simulink model "ex1"  (R2015a)
settings: Solver=ode45  StartTime=0.0  StopTime=10.0  RelTol=1e-3
values from neighbouring files (symbols this model uses):
  Nfft = 128    [e1.m]
  Ng = 16    [e1.m]
  Nsym = Nfft+Ng    (= 144)    [e1.m]
undefined symbols (not defined in the file or in its folder): get, magnitude
libraries: dspxfrm3 x2, dspindex x2, commdigbbndam3 x2, dspsnks4 x2, dspstat3 x2, commchan3 x1, commrandsrc2 x1, commsink2 x1, simulink x1
settings Model: Creator=david  LastModifiedBy=ctu

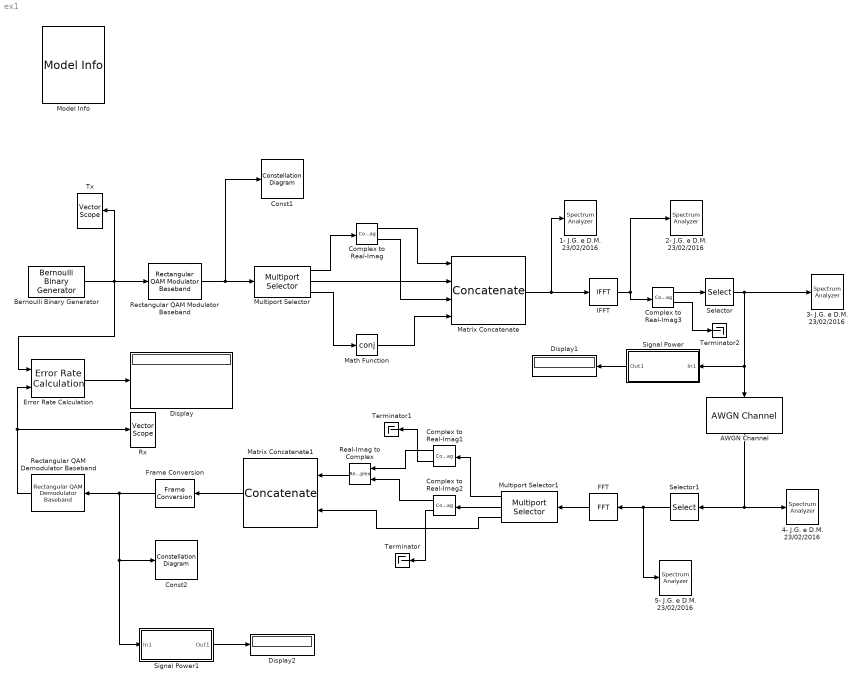
== system ex1 ==
  1- J.G. e D.M. 23/02/2016 : SpectrumAnalyzer
  2- J.G. e D.M. 23/02/2016 : SpectrumAnalyzer
  3- J.G. e D.M. 23/02/2016 : SpectrumAnalyzer
  4- J.G. e D.M. 23/02/2016 : SpectrumAnalyzer
  5- J.G. e D.M. 23/02/2016 : SpectrumAnalyzer
  AWGN Channel : commchan3/AWGN Channel  InputProcessing=Columns as channels (frame based)  seed=67  noiseMode="Signal to noise ratio  (Eb/No)"  EbNodB=8  EsNodB=10  SNRdB=10  bitsPerSym=Nblock  Ps=1/Nfft  Tsym=Tsym  variance=1
  Bernoulli Binary Generator : commrandsrc2/Bernoulli Binary Generator  P=0.5  seed=61  Ts=Tsym/Nblock  frameBased=on  sampPerFrame=Nblock  orient=off  outDataType=double
  Complex to Real-Imag{,1..3} (4 alike) : ComplexToRealImag
  Const1 : ConstellationDiagram
  Const2 : ConstellationDiagram
  Display : Display
      settings: Format=short_e
  Display1 : Display
  Display2 : Display
  Error Rate Calculation : commsink2/Error Rate Calculation  N=0  st_delay=0  cp_mode=Entire frame  subframe=[]  PMode=Port  WsName=ErrorVec  RsMode2=off  stop=on  numErr=100  maxBits=1e6
  FFT : dspxfrm3/FFT  CompMethod=Table lookup  TableOpt=NEW  TableOptActive=Speed  BitRevOrder=off  InheritFFTLength=on  FFTLength=64  WrapInput=on  RowConvenienceOn=on  FFTImplementation=Auto  SkipNorm=off  firstCoeffDataTypeStr=Inherit: Same word length as input  firstCoeffLastDataTypeStr=Inherit: Same word length as input  outputMin=[]  outputMax=[]  roundingMode=Floor  overflowMode=off
  Frame Conversion : FrameConversion
  IFFT : dspxfrm3/IFFT  CompMethod=Table lookup  TableOpt=NEW  TableOptActive=Speed  BitRevOrder=off  cs_in=off  SkipNorm=on  InheritFFTLength=on  FFTLength=64  WrapInput=on  mode=Complex  outSamplingMode=Sample based  RowConvenienceOn=on  FFTImplementation=Auto  firstCoeffDataTypeStr=Inherit: Same word length as input  firstCoeffLastDataTypeStr=Inherit: Same word length as input  outputMin=[]  outputMax=[]  roundingMode=Floor  overflowMode=off
  Math Function : Math  Operator=conj  SaturateOnIntegerOverflow=on
  Matrix Concatenate : Concatenate  NumInputs=4  Mode=Multidimensional array
  Matrix Concatenate1 : Concatenate  Mode=Multidimensional array
  Model Info : simulink/Model-Wide Utilities/Model Info  Frame=on  DisplayStringWithTags=|  HorizontalTextAlignment=Center  LeftAlignmentValue=0.5  SourceBlockDiagram=ex1  TagMaxNumber=20
      | b=4; 
      | M=2^b;
      | Nfft=128; 
      | Nffth=Nfft/2;
      | Nblock=Nffth*b;
      | Ng = 16; 
      | Nsym= Nfft+Ng;
      | Tsym=0.001;
      | SNRbdB=10;
  Multiport Selector : dspindex/Multiport Selector  rowsOrCols=Rows  idxCellArray={ 1, 2:Nffth, Nffth:-1:2}  idxErrMode=Clip Index
  Multiport Selector1 : dspindex/Multiport Selector  rowsOrCols=Rows  idxCellArray={ 1, Nffth+1, 2:Nffth}  idxErrMode=Clip Index
  Real-Imag to Complex : RealImagToComplex
  Rectangular QAM Demodulator Baseband : commdigbbndam3/Rectangular QAM Demodulator Baseband  M=M  PowType=Average Power  MinDist=2  AvgPow=1  PeakPow=1  Ph=0  Dec=Gray  Mapping=[0:15]  OutType=Bit  DecType=Hard decision  VarSource=Dialog  Variance=1  outDtype1=Inherit via internal rule  outDtype2=Inherit via internal rule  derotateFactorWordLen=16  denormFactorWordLen=16  prodOutWordLen=32  prodOutRoundingMode=Floor  prodOutOverflowMode=Wrap  sumWordLen=32
  Rectangular QAM Modulator Baseband : commdigbbndam3/Rectangular QAM Modulator Baseband  M=M  InType=Bit  Enc=Gray  Mapping=[0:15]  PowType=Average Power  MinDist=2  AvgPow=1  PeakPow=1  Ph=0  outDtype=double  outWordLen=16  outUDDataType=sfix(16)  outFracLenMode=Best precision  outFracLen=15
  Rx : dspsnks4/Vector Scope  ScopeProperties=on  Domain=Time  HorizSpan=1  DisplayProperties=off  AxisGrid=on  Memory=off  FrameNumber=on  AxisLegend=off  AxisZoom=off  OpenScopeAtSimStart=on  OpenScopeImmediately=off  FigPos=get(0,'defaultfigureposition')  AxisProperties=off  XUnits=Hertz  XRange=[0...Fs/2]  InheritXIncr=on  XIncr=1  XLabel=Time  XLimit=Auto  XMin=0  XMax=1  XStart=0  YUnits=dB  YLabel=Amplitude  LineProperties=off  XAxisParamsVer=6.9
      settings: YMin=-10  YMax=10
  Selector : Selector  InputPortWidth=Nfft  Indices=[Nfft-Ng+1:Nfft 1:Nfft]
  Selector1 : Selector  InputPortWidth=Nsym  Indices=[Ng+1:Nsym]
  Signal Power : Subsystem
  Signal Power1 : Subsystem
  Terminator : Terminator
  Terminator1 : Terminator
  Terminator2 : Terminator
  Tx : dspsnks4/Vector Scope  ScopeProperties=on  Domain=Time  HorizSpan=1  DisplayProperties=off  AxisGrid=on  Memory=off  FrameNumber=on  AxisLegend=off  AxisZoom=off  OpenScopeAtSimStart=on  OpenScopeImmediately=off  FigPos=get(0,'defaultfigureposition')  AxisProperties=off  XUnits=Hertz  XRange=[0...Fs/2]  InheritXIncr=on  XIncr=1  XLabel=Time  XLimit=Auto  XMin=0  XMax=1  XStart=0  YUnits=dB  YLabel=Amplitude  LineProperties=off  XAxisParamsVer=6.9
      settings: YMin=-10  YMax=10
  wires:
  Bernoulli Binary Generator/1 -> Tx/1, Error Rate Calculation/1, Rectangular QAM Modulator Baseband/1
  Rectangular QAM Modulator Baseband/1 -> Const1/1, Multiport Selector/1
  Multiport Selector/1 -> Complex to Real-Imag/1
  Multiport Selector/3 -> Math Function/1
  Complex to Real-Imag/1 -> Matrix Concatenate/1
  Multiport Selector/2 -> Matrix Concatenate/2
  Complex to Real-Imag/2 -> Matrix Concatenate/3
  Math Function/1 -> Matrix Concatenate/4
  Matrix Concatenate/1 -> 1- J.G. e D.M. 23/02/2016/1, IFFT/1
  IFFT/1 -> Complex to Real-Imag3/1, 2- J.G. e D.M. 23/02/2016/1
  Selector/1 -> 3- J.G. e D.M. 23/02/2016/1, Signal Power/1(In1), AWGN Channel/1
  AWGN Channel/1 -> Selector1/1, 4- J.G. e D.M. 23/02/2016/1
  Selector1/1 -> 5- J.G. e D.M. 23/02/2016/1, FFT/1
  FFT/1 -> Multiport Selector1/1
  Multiport Selector1/1 -> Complex to Real-Imag1/1
  Multiport Selector1/2 -> Complex to Real-Imag2/1
  Complex to Real-Imag1/1 -> Real-Imag to Complex/1
  Complex to Real-Imag2/1 -> Real-Imag to Complex/2
  Real-Imag to Complex/1 -> Matrix Concatenate1/1
  Multiport Selector1/3 -> Matrix Concatenate1/2
  Matrix Concatenate1/1 -> Frame Conversion/1
  Frame Conversion/1 -> Const2/1, Signal Power1/1(In1), Rectangular QAM Demodulator Baseband/1
  Rectangular QAM Demodulator Baseband/1 -> Rx/1, Error Rate Calculation/2
  Error Rate Calculation/1 -> Display/1
  Signal Power/1(Out1) -> Display1/1
  Signal Power1/1(Out1) -> Display2/1
  Complex to Real-Imag1/2 -> Terminator1/1
  Complex to Real-Imag2/2 -> Terminator/1
  Complex to Real-Imag3/1 -> Selector/1
  Complex to Real-Imag3/2 -> Terminator2/1

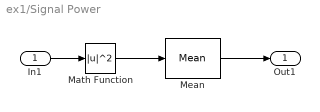
== system ex1/Signal Power ==
  In1 : Inport
  Math Function : Math  Operator=magnitude^2  SaturateOnIntegerOverflow=on
  Mean : dspstat3/Mean  run=on  reset_popup=None  InputProcessing=Columns as channels (frame based)  directionMode=Each column  dimension=1  treatSBRowAsCol=off  roiEnable=off  roiType=Rectangles  roiPortion=Entire ROI  roiOutput=Individual statistics for each ROI  roiFlag=off  outputDataTypeStr=Inherit: Same as accumulator  outputLastDataTypeStr=Inherit: Same as accumulator  outputMin=[]  outputMax=[]  roundingMode=Floor  overflowMode=off
  Out1 : Outport
  wires:
  In1/1 -> Math Function/1
  Math Function/1 -> Mean/1
  Mean/1 -> Out1/1

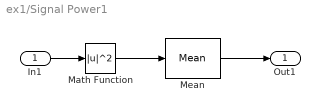
== system ex1/Signal Power1 ==
  In1 : Inport
  Math Function : Math  Operator=magnitude^2  SaturateOnIntegerOverflow=on
  Mean : dspstat3/Mean  run=on  reset_popup=None  InputProcessing=Columns as channels (frame based)  directionMode=Each column  dimension=1  treatSBRowAsCol=off  roiEnable=off  roiType=Rectangles  roiPortion=Entire ROI  roiOutput=Individual statistics for each ROI  roiFlag=off  outputDataTypeStr=Inherit: Same as accumulator  outputLastDataTypeStr=Inherit: Same as accumulator  outputMin=[]  outputMax=[]  roundingMode=Floor  overflowMode=off
  Out1 : Outport
  wires:
  In1/1 -> Math Function/1
  Math Function/1 -> Mean/1
  Mean/1 -> Out1/1
